simulink model "drones_simulation"  (R2025b)
settings: Solver=ode4  StartTime=0.0  StopTime=t_sim  FixedStep=Ts  RelTol=1e-3
values from neighbouring files (symbols this model uses):
  adj_row_1 = Adj_mat(1,:)    [Parameters_scenarios.m]
  adj_row_2 = Adj_mat(2,:)    [Parameters_scenarios.m]
  adj_row_3 = Adj_mat(3,:)    [Parameters_scenarios.m]
  adj_row_4 = Adj_mat(4,:)    [Parameters_scenarios.m]
  gamma1 = 8.0    (= 8)    [Parameters_scenarios.m]
  gamma2 = 8.0    (= 8)    [Parameters_scenarios.m]
  goal_tolerance = 0.05    [Parameters_scenarios.m]
  Ib = diag([Jxx, Jyy, Jzz])    [Parameters_scenarios.m]
  Kd = 2.5    [Parameters_scenarios.m]
  Kp = 1.2    [Parameters_scenarios.m]
  mass = 0.032    [Parameters_scenarios.m]
  max_acc = 2.5    [Parameters_scenarios.m]
  max_vel = 1.2 * (dist_total / desired_flight_time)    [Parameters_scenarios.m]
  Rc = 2.0    (= 2)    [Parameters_scenarios.m]
  Rs = Rs_safe    (= 0.15)    [Parameters_scenarios.m]
  Rs_obs = radius_robots + radii_obstacles + margin    (= 0.95)    [Parameters_scenarios.m]
  v0_1 = v0(1,:)'    [Parameters_scenarios.m]
  v0_2 = v0(2,:)'    [Parameters_scenarios.m]
  v0_3 = v0(3,:)'    [Parameters_scenarios.m]
  v0_4 = v0(4,:)'    [Parameters_scenarios.m]
  x0_1 = x0(1,:)'    [Parameters_scenarios.m]
  x0_2 = x0(2,:)'    [Parameters_scenarios.m]
  x0_3 = x0(3,:)'    [Parameters_scenarios.m]
  x0_4 = x0(4,:)'    [Parameters_scenarios.m]
  x_objects = [0.0 ... (first row only)    [Parameters_scenarios.m]
  xg_1 = xg(1,:)'    [Parameters_scenarios.m]
  xg_2 = xg(2,:)'    [Parameters_scenarios.m]
  xg_3 = xg(3,:)'    [Parameters_scenarios.m]
  xg_4 = xg(4,:)'    [Parameters_scenarios.m]
  xg_vec = reshape(xg', [], 1)    [Parameters_scenarios.m]
libraries: robotcorelib x4
(part 1 of 3)
settings Model: Creator=aless  LastModifiedBy=Alessia

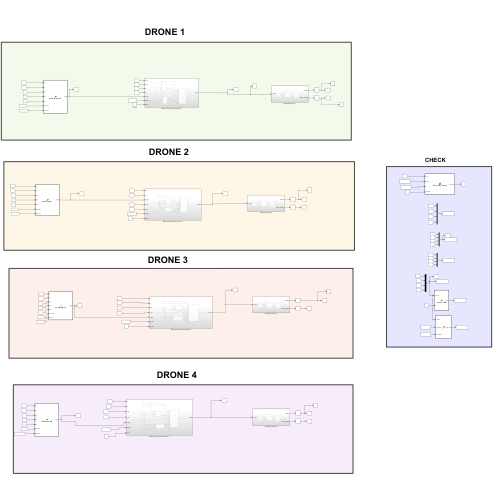
[thumbnail: Simulink's stored preview of the top-level diagram]
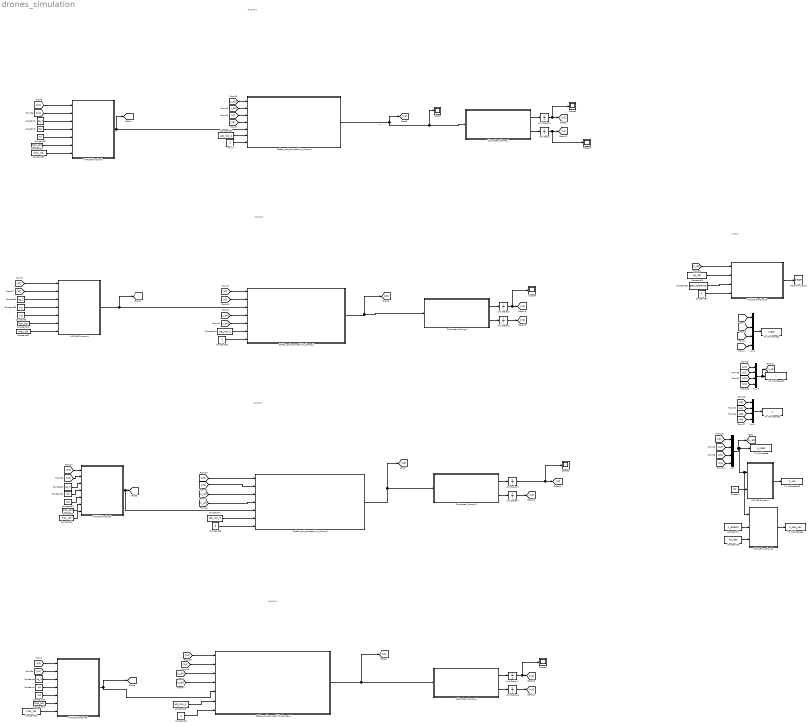
== system drones_simulation ==
  note: DRONE 1
  note: a
  note: DRONE 2
  note: DRONE 3
  note: DRONE 4
  note: CHECK
  Constant : Constant  Value=Rs
  Constant1 : Constant  Value=xg_1
  Constant17 : Constant  Value=x_objects
  Constant18 : Constant  Value=Rs_obs
  Constant2 : Constant  Value=xg_2
  Constant{6,27,32..33} (4 alike) : Constant  Value=Kd
  Constant{5,28..29,34} (4 alike) : Constant  Value=max_acc
  Constant3 : Constant  Value=xg_3
  Constant{4,7,30..31} (4 alike) : Constant  Value=Kp
  Constant47 : Constant  Value=adj_row_3
  Constant48 : Constant  Value=adj_row_4
  Constant49 : Constant  Value=adj_row_2
  Constant50 : Constant  Value=adj_row_1
  Constant52 : Constant  Value=2
  Constant53 : Constant  Value=3
  Constant54 : Constant  Value=4
  Constant{59..62} (4 alike) : Constant  Value=max_vel
  Constant63 : Constant  Value=goal_tolerance
  Constant64 : Constant  Value=4
  Constant65 : Constant  Value=xg_vec
  Constant8 : Constant  Value=xg_4
  MATLAB Function : MATLAB Function  TreatAsAtomicUnit=on
  MATLAB Function13 : MATLAB Function  TreatAsAtomicUnit=on
  MATLAB Function18 : MATLAB Function  TreatAsAtomicUnit=on
  MATLAB Function3 : MATLAB Function  TreatAsAtomicUnit=on
  MATLAB Function4 : MATLAB Function  TreatAsAtomicUnit=on
  MATLAB Function5 : MATLAB Function  TreatAsAtomicUnit=on
  MATLAB Function6 : MATLAB Function  TreatAsAtomicUnit=on
  Mux{,1..3} (4 alike) : Mux
  Safety_and_connectivity_Drone_1 : Subsystem
  Safety_and_connectivity_Drone_2 : Subsystem
  Safety_and_connectivity_Drone_3 : Subsystem
  Safety_and_connectivity_Drone_4 : Subsystem
  Scope{,3..7} (6 alike) : Scope
      Scope settings: ActiveDisplayYMinimum=-0.97415805527828381  ActiveDisplayYMaximum=3.2901969224528962
      Scope3 settings: ActiveDisplayYMinimum=-0.78272111630723207  ActiveDisplayYMaximum=1.9854335134906034  DataLoggingVariableName=ScopeData7
      Scope4 settings: ActiveDisplayYMinimum=-0.46546142132174678  ActiveDisplayYMaximum=0.18915279189572098  DataLoggingVariableName=ScopeData8
      Scope5 settings: ActiveDisplayYMinimum=-0.57335527047203139  ActiveDisplayYMaximum=1.160197434248283  DataLoggingVariableName=ScopeData9
      Scope6 settings: ActiveDisplayYMinimum=-0.5009829844423257  ActiveDisplayYMaximum=1.5088468599809324  DataLoggingVariableName=ScopeData10
      Scope7 settings: ActiveDisplayYMinimum=-0.78272111630723207  ActiveDisplayYMaximum=1.9854335134906034  DataLoggingVariableName=ScopeData12
  Stop Simulation : Stop
  Subsystem_Drone_1 : Subsystem
  Subsystem_Drone_2 : Subsystem
  Subsystem_Drone_3 : Subsystem
  Subsystem_Drone_4 : Subsystem
  To Workspace : ToWorkspace  VariableName=x_robot  SaveFormat=Timeseries  SampleTime=-1
  To Workspace1 : ToWorkspace  VariableName=u  SaveFormat=Timeseries  SampleTime=-1
  To Workspace2 : ToWorkspace  VariableName=u_gtg  SaveFormat=Timeseries  SampleTime=-1
  To Workspace3 : ToWorkspace  VariableName=h_vec  SaveFormat=Timeseries  SampleTime=-1
  To Workspace4 : ToWorkspace  VariableName=h_obs_vec  SaveFormat=Timeseries  SampleTime=-1
  To Workspace5 : ToWorkspace  VariableName=v  SaveFormat=Timeseries  SampleTime=-1
  Unit Delay{,1..7} (8 alike) : UnitDelay  SampleTime=-1  HasFrameUpgradeWarning=on
  my_id : Constant
  wires:
  [x4] -> Mux/4
  [x2] -> Mux/2
  [x4] -> MATLAB Function6/1(x_i)
  [x2] -> MATLAB Function4/1(x_i)
  Constant2/1 -> MATLAB Function4/3(xg_i)
  MATLAB Function/1(h_vec) -> To Workspace3/1
  Constant3/1 -> MATLAB Function5/3(xg_i)
  Mux1/1 -> To Workspace1/1
  Constant1/1 -> MATLAB Function3/3(xg_i)
  Mux/1 -> [x_all], To Workspace/1, MATLAB Function13/1(x_robot), MATLAB Function/1(x_robot)
  [x1] -> MATLAB Function3/1(x_i)
  [x1] -> Mux/1
  [u2] -> Mux1/2
  [x3] -> MATLAB Function5/1(x_i)
  [x3] -> Mux/3
  [u1] -> Mux1/1
  [u4] -> Mux1/4
  Constant/1 -> MATLAB Function/2(Rs)
  Constant8/1 -> MATLAB Function6/3(xg_i)
  [u3] -> Mux1/3
  Constant18/1 -> MATLAB Function13/3(Rs_objects)
  MATLAB Function13/1(h_obs_vec) -> To Workspace4/1
  Constant17/1 -> MATLAB Function13/2(x_objects)
  [u_gtg1] -> Mux2/1
  [u_gtg2] -> Mux2/2
  [u_gtg3] -> Mux2/3
  [u_gtg4] -> Mux2/4
  Mux2/1 -> To Workspace2/1
  [v3] -> Mux3/3
  Mux3/1 -> [v_all], To Workspace5/1
  [v1] -> Mux3/1
  [v2] -> Mux3/2
  [v4] -> Mux3/4
  [v1] -> MATLAB Function3/2(v_i)
  Constant7/1 -> MATLAB Function3/4(Kp)
  Constant27/1 -> MATLAB Function3/5(Kd)
  Constant28/1 -> MATLAB Function3/6(max_acc)
  [v2] -> MATLAB Function4/2(v_i)
  Constant29/1 -> MATLAB Function4/6(max_acc)
  Constant6/1 -> MATLAB Function4/5(Kd)
  Constant30/1 -> MATLAB Function4/4(Kp)
  [v3] -> MATLAB Function5/2(v_i)
  Constant31/1 -> MATLAB Function5/4(Kp)
  Constant32/1 -> MATLAB Function5/5(Kd)
  Constant5/1 -> MATLAB Function5/6(max_acc)
  Constant34/1 -> MATLAB Function6/6(max_acc)
  Constant33/1 -> MATLAB Function6/5(Kd)
  Constant4/1 -> MATLAB Function6/4(Kp)
  [v4] -> MATLAB Function6/2(v_i)
  MATLAB Function6/1(u_gtg) -> [u_gtg4], Safety_and_connectivity_Drone_4/5(u_gtg)
  MATLAB Function4/1(u_gtg) -> [u_gtg2], Safety_and_connectivity_Drone_2/3(u_gtg)
  Subsystem_Drone_1/1(Position) -> Unit Delay1/1
  Subsystem_Drone_1/2(Linear_velocity) -> Unit Delay/1
  Unit Delay1/1 -> Scope3/1, [x1]
  Unit Delay/1 -> Scope7/1, [v1]
  Unit Delay2/1 -> [v2]
  Subsystem_Drone_2/2(Linear_velocity) -> Unit Delay2/1
  Subsystem_Drone_2/1(Position) -> Unit Delay3/1
  Unit Delay4/1 -> [v3]
  Subsystem_Drone_3/2(Linear_velocity) -> Unit Delay4/1
  Subsystem_Drone_3/1(Position) -> Unit Delay5/1
  Unit Delay6/1 -> [v4]
  Subsystem_Drone_4/2(Linear_velocity) -> Unit Delay6/1
  Subsystem_Drone_4/1(Position) -> Unit Delay7/1
  Unit Delay3/1 -> Scope4/1, [x2]
  Unit Delay5/1 -> Scope5/1, [x3]
  Unit Delay7/1 -> Scope6/1, [x4]
  Constant59/1 -> MATLAB Function3/7(max_vel)
  Constant60/1 -> MATLAB Function4/7(max_vel)
  Constant61/1 -> MATLAB Function5/7(max_vel)
  Constant62/1 -> MATLAB Function6/7(max_vel)
  MATLAB Function18/1(stop_sim) -> Stop Simulation/1
  [x_all] -> MATLAB Function18/1(x_all)
  Constant63/1 -> MATLAB Function18/3(tol)
  Constant64/1 -> MATLAB Function18/4(n_robots)
  Constant65/1 -> MATLAB Function18/2(xg_vec)
  Safety_and_connectivity_Drone_1/1(u_safe) -> [u1], Scope/1, Subsystem_Drone_1/1(u_safe)
  MATLAB Function3/1(u_gtg) -> [u_gtg1], Safety_and_connectivity_Drone_1/5(u_gtg)
  Constant50/1 -> Safety_and_connectivity_Drone_1/6(adj_row)
  my_id/1 -> Safety_and_connectivity_Drone_1/7(my_id)
  [x_all] -> Safety_and_connectivity_Drone_1/1(x_all)
  [v_all] -> Safety_and_connectivity_Drone_1/2(v_all)
  [x1] -> Safety_and_connectivity_Drone_1/3(x_i)
  [v1] -> Safety_and_connectivity_Drone_1/4(v_i)
  Safety_and_connectivity_Drone_2/1(u_safe) -> [u2], Subsystem_Drone_2/1(u_safe)
  [x2] -> Safety_and_connectivity_Drone_2/1(x_i)
  [v2] -> Safety_and_connectivity_Drone_2/2(v_i)
  [x_all] -> Safety_and_connectivity_Drone_2/4(x_all)
  [v_all] -> Safety_and_connectivity_Drone_2/5(v_all)
  Constant49/1 -> Safety_and_connectivity_Drone_2/6(adj_row)
  Constant52/1 -> Safety_and_connectivity_Drone_2/7(my_id)
  Safety_and_connectivity_Drone_3/1(u_safe) -> [u3], Subsystem_Drone_3/1(u_safe)
  [x3] -> Safety_and_connectivity_Drone_3/1(x_i)
  [v3] -> Safety_and_connectivity_Drone_3/2(v_i)
  [x_all] -> Safety_and_connectivity_Drone_3/3(x_all)
  [v_all] -> Safety_and_connectivity_Drone_3/4(v_all)
  MATLAB Function5/1(u_gtg) -> Safety_and_connectivity_Drone_3/5(u_gtg), [u_gtg3]
  Constant47/1 -> Safety_and_connectivity_Drone_3/6(adj_row)
  Constant53/1 -> Safety_and_connectivity_Drone_3/7(my_id)
  Safety_and_connectivity_Drone_4/1(u_safe) -> [u4], Subsystem_Drone_4/1(u_safe)
  [x4] -> Safety_and_connectivity_Drone_4/1(x_i)
  [v4] -> Safety_and_connectivity_Drone_4/2(v_i)
  [x_all] -> Safety_and_connectivity_Drone_4/3(x_all)
  [v_all] -> Safety_and_connectivity_Drone_4/4(v_all)
  Constant48/1 -> Safety_and_connectivity_Drone_4/6(adj_row)
  Constant54/1 -> Safety_and_connectivity_Drone_4/7(my_id)

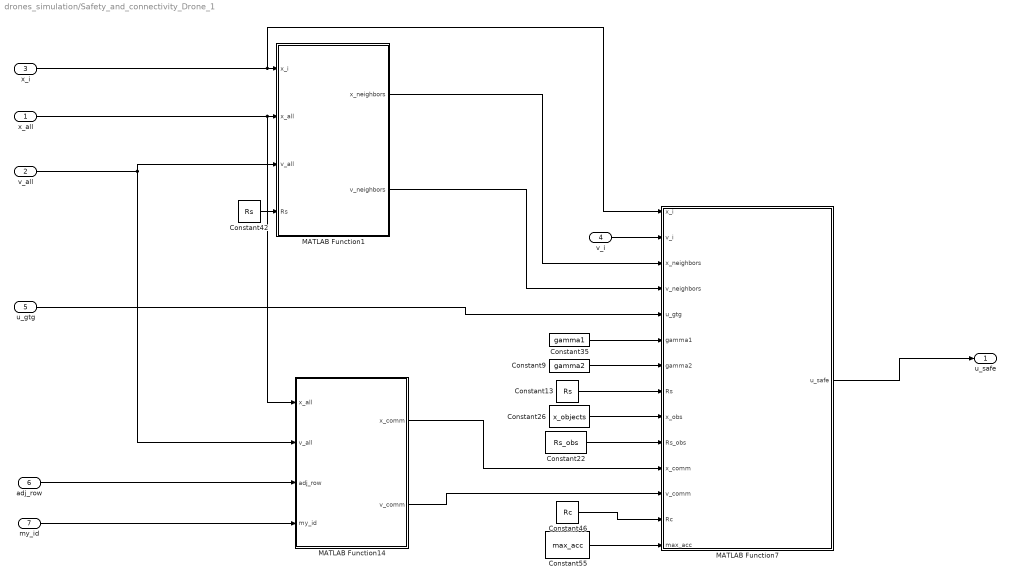
== system drones_simulation/Safety_and_connectivity_Drone_1 ==
  x_all : Inport
  v_all : Inport  Port=2
  x_i : Inport  Port=3
  v_i : Inport  Port=4
  u_gtg : Inport  Port=5
  adj_row : Inport  Port=6
  my_id : Inport  Port=7
  Constant13 : Constant  Value=Rs
  Constant22 : Constant  Value=Rs_obs
  Constant26 : Constant  Value=x_objects
  Constant35 : Constant  Value=gamma1
  Constant42 : Constant  Value=Rs
  Constant46 : Constant  Value=Rc
  Constant55 : Constant  Value=max_acc
  Constant9 : Constant  Value=gamma2
  MATLAB Function1 : MATLAB Function  TreatAsAtomicUnit=on
  MATLAB Function14 : MATLAB Function  TreatAsAtomicUnit=on
  MATLAB Function7 : MATLAB Function  TreatAsAtomicUnit=on
  u_safe : Outport
  wires:
  Constant35/1 -> MATLAB Function7/6(gamma1)
  Constant42/1 -> MATLAB Function1/4(Rs)
  u_gtg/1 -> MATLAB Function7/5(u_gtg)
  Constant22/1 -> MATLAB Function7/10(Rs_obs)
  Constant26/1 -> MATLAB Function7/9(x_obs)
  Constant55/1 -> MATLAB Function7/14(max_acc)
  MATLAB Function1/2(v_neighbors) -> MATLAB Function7/4(v_neighbors)
  MATLAB Function14/2(v_comm) -> MATLAB Function7/12(v_comm)
  MATLAB Function1/1(x_neighbors) -> MATLAB Function7/3(x_neighbors)
  MATLAB Function14/1(x_comm) -> MATLAB Function7/11(x_comm)
  Constant13/1 -> MATLAB Function7/8(Rs)
  x_all/1 -> MATLAB Function14/1(x_all), MATLAB Function1/2(x_all)
  Constant46/1 -> MATLAB Function7/13(Rc)
  Constant9/1 -> MATLAB Function7/7(gamma2)
  v_all/1 -> MATLAB Function1/3(v_all), MATLAB Function14/2(v_all)
  adj_row/1 -> MATLAB Function14/3(adj_row)
  MATLAB Function7/1(u_safe) -> u_safe/1
  my_id/1 -> MATLAB Function14/4(my_id)
  x_i/1 -> MATLAB Function7/1(x_i), MATLAB Function1/1(x_i)
  v_i/1 -> MATLAB Function7/2(v_i)

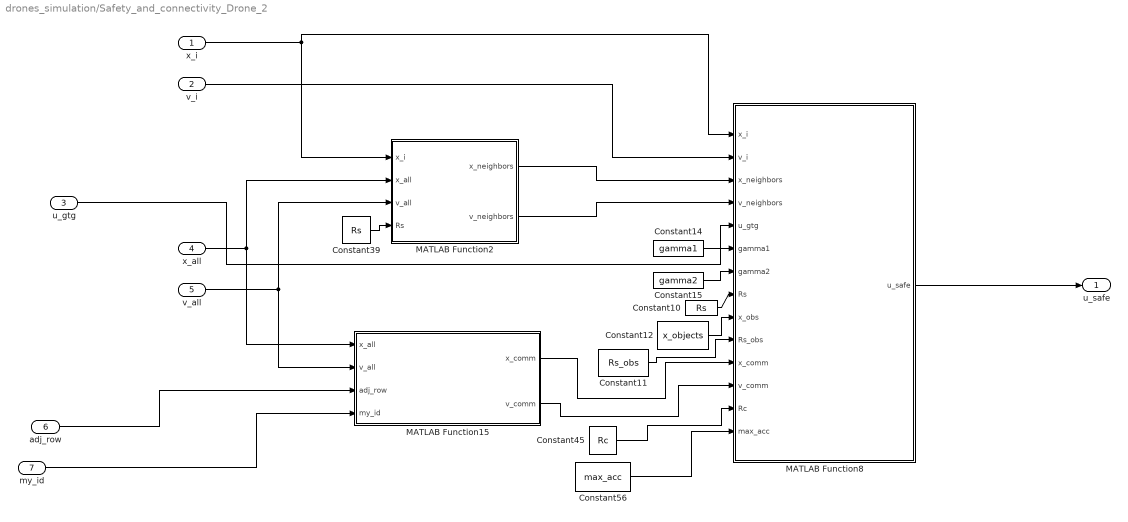
== system drones_simulation/Safety_and_connectivity_Drone_2 ==
  x_i : Inport
  v_i : Inport  Port=2
  u_gtg : Inport  Port=3
  x_all : Inport  Port=4
  v_all : Inport  Port=5
  adj_row : Inport  Port=6
  my_id : Inport  Port=7
  Constant10 : Constant  Value=Rs
  Constant11 : Constant  Value=Rs_obs
  Constant12 : Constant  Value=x_objects
  Constant14 : Constant  Value=gamma1
  Constant15 : Constant  Value=gamma2
  Constant39 : Constant  Value=Rs
  Constant45 : Constant  Value=Rc
  Constant56 : Constant  Value=max_acc
  MATLAB Function15 : MATLAB Function  TreatAsAtomicUnit=on
  MATLAB Function2 : MATLAB Function  TreatAsAtomicUnit=on
  MATLAB Function8 : MATLAB Function  TreatAsAtomicUnit=on
  u_safe : Outport
  wires:
  MATLAB Function2/2(v_neighbors) -> MATLAB Function8/4(v_neighbors)
  Constant39/1 -> MATLAB Function2/4(Rs)
  Constant45/1 -> MATLAB Function8/13(Rc)
  MATLAB Function2/1(x_neighbors) -> MATLAB Function8/3(x_neighbors)
  MATLAB Function15/2(v_comm) -> MATLAB Function8/12(v_comm)
  MATLAB Function15/1(x_comm) -> MATLAB Function8/11(x_comm)
  x_i/1 -> MATLAB Function2/1(x_i), MATLAB Function8/1(x_i)
  Constant10/1 -> MATLAB Function8/8(Rs)
  Constant15/1 -> MATLAB Function8/7(gamma2)
  Constant12/1 -> MATLAB Function8/9(x_obs)
  v_all/1 -> MATLAB Function15/2(v_all), MATLAB Function2/3(v_all)
  Constant14/1 -> MATLAB Function8/6(gamma1)
  Constant11/1 -> MATLAB Function8/10(Rs_obs)
  Constant56/1 -> MATLAB Function8/14(max_acc)
  x_all/1 -> MATLAB Function15/1(x_all), MATLAB Function2/2(x_all)
  adj_row/1 -> MATLAB Function15/3(adj_row)
  u_gtg/1 -> MATLAB Function8/5(u_gtg)
  my_id/1 -> MATLAB Function15/4(my_id)
  v_i/1 -> MATLAB Function8/2(v_i)
  MATLAB Function8/1(u_safe) -> u_safe/1

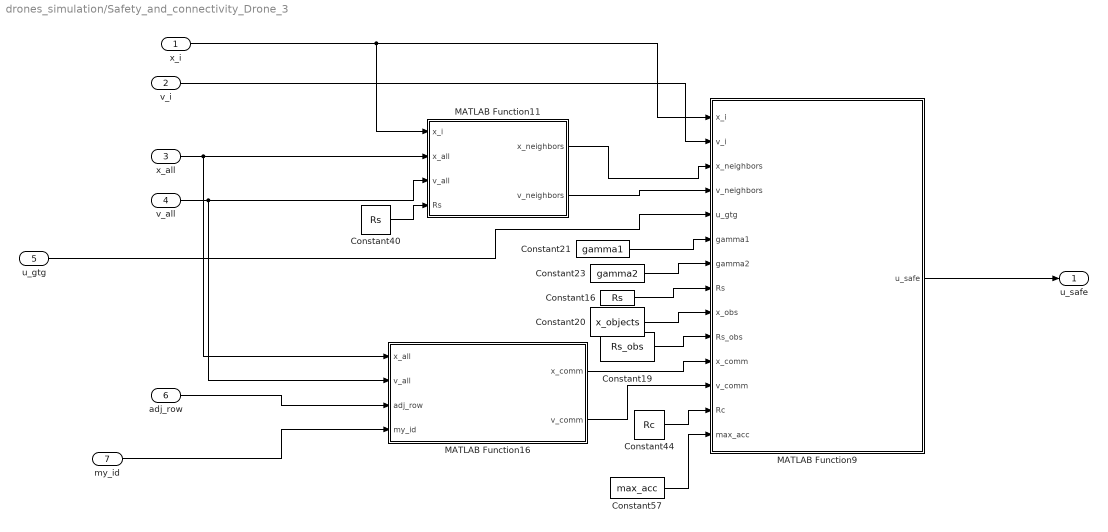
== system drones_simulation/Safety_and_connectivity_Drone_3 ==
  x_i : Inport
  v_i : Inport  Port=2
  x_all : Inport  Port=3
  v_all : Inport  Port=4
  u_gtg : Inport  Port=5
  adj_row : Inport  Port=6
  my_id : Inport  Port=7
  Constant16 : Constant  Value=Rs
  Constant19 : Constant  Value=Rs_obs
  Constant20 : Constant  Value=x_objects
  Constant21 : Constant  Value=gamma1
  Constant23 : Constant  Value=gamma2
  Constant40 : Constant  Value=Rs
  Constant44 : Constant  Value=Rc
  Constant57 : Constant  Value=max_acc
  MATLAB Function11 : MATLAB Function  TreatAsAtomicUnit=on
  MATLAB Function16 : MATLAB Function  TreatAsAtomicUnit=on
  MATLAB Function9 : MATLAB Function  TreatAsAtomicUnit=on
  u_safe : Outport
  wires:
  MATLAB Function11/2(v_neighbors) -> MATLAB Function9/4(v_neighbors)
  v_all/1 -> MATLAB Function11/3(v_all), MATLAB Function16/2(v_all)
  MATLAB Function16/1(x_comm) -> MATLAB Function9/11(x_comm)
  Constant20/1 -> MATLAB Function9/9(x_obs)
  Constant16/1 -> MATLAB Function9/8(Rs)
  v_i/1 -> MATLAB Function9/2(v_i)
  Constant40/1 -> MATLAB Function11/4(Rs)
  Constant23/1 -> MATLAB Function9/7(gamma2)
  u_gtg/1 -> MATLAB Function9/5(u_gtg)
  Constant57/1 -> MATLAB Function9/14(max_acc)
  Constant21/1 -> MATLAB Function9/6(gamma1)
  MATLAB Function11/1(x_neighbors) -> MATLAB Function9/3(x_neighbors)
  x_all/1 -> MATLAB Function11/2(x_all), MATLAB Function16/1(x_all)
  Constant44/1 -> MATLAB Function9/13(Rc)
  Constant19/1 -> MATLAB Function9/10(Rs_obs)
  MATLAB Function16/2(v_comm) -> MATLAB Function9/12(v_comm)
  x_i/1 -> MATLAB Function9/1(x_i), MATLAB Function11/1(x_i)
  adj_row/1 -> MATLAB Function16/3(adj_row)
  my_id/1 -> MATLAB Function16/4(my_id)
  MATLAB Function9/1(u_safe) -> u_safe/1

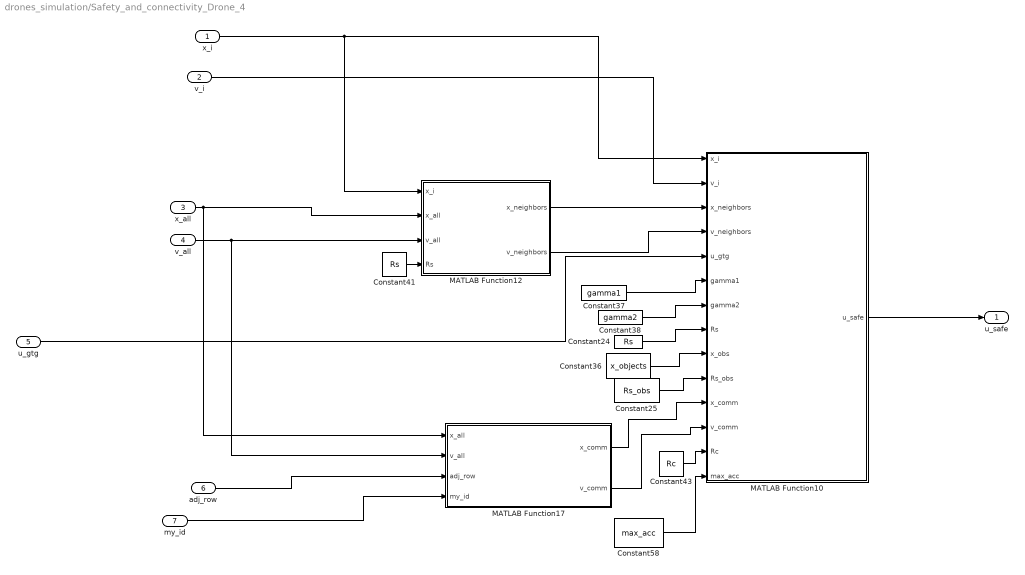
== system drones_simulation/Safety_and_connectivity_Drone_4 ==
  x_i : Inport
  v_i : Inport  Port=2
  x_all : Inport  Port=3
  v_all : Inport  Port=4
  u_gtg : Inport  Port=5
  adj_row : Inport  Port=6
  my_id : Inport  Port=7
  Constant24 : Constant  Value=Rs
  Constant25 : Constant  Value=Rs_obs
  Constant36 : Constant  Value=x_objects
  Constant37 : Constant  Value=gamma1
  Constant38 : Constant  Value=gamma2
  Constant41 : Constant  Value=Rs
  Constant43 : Constant  Value=Rc
  Constant58 : Constant  Value=max_acc
  MATLAB Function10 : MATLAB Function  TreatAsAtomicUnit=on
  MATLAB Function12 : MATLAB Function  TreatAsAtomicUnit=on
  MATLAB Function17 : MATLAB Function  TreatAsAtomicUnit=on
  u_safe : Outport
  wires:
  x_all/1 -> MATLAB Function17/1(x_all), MATLAB Function12/2(x_all)
  MATLAB Function12/2(v_neighbors) -> MATLAB Function10/4(v_neighbors)
  Constant58/1 -> MATLAB Function10/14(max_acc)
  Constant25/1 -> MATLAB Function10/10(Rs_obs)
  adj_row/1 -> MATLAB Function17/3(adj_row)
  Constant38/1 -> MATLAB Function10/7(gamma2)
  Constant43/1 -> MATLAB Function10/13(Rc)
  MATLAB Function12/1(x_neighbors) -> MATLAB Function10/3(x_neighbors)
  MATLAB Function17/1(x_comm) -> MATLAB Function10/11(x_comm)
  MATLAB Function17/2(v_comm) -> MATLAB Function10/12(v_comm)
  Constant36/1 -> MATLAB Function10/9(x_obs)
  Constant37/1 -> MATLAB Function10/6(gamma1)
  Constant41/1 -> MATLAB Function12/4(Rs)
  u_gtg/1 -> MATLAB Function10/5(u_gtg)
  Constant24/1 -> MATLAB Function10/8(Rs)
  x_i/1 -> MATLAB Function10/1(x_i), MATLAB Function12/1(x_i)
  v_all/1 -> MATLAB Function17/2(v_all), MATLAB Function12/3(v_all)
  MATLAB Function10/1(u_safe) -> u_safe/1
  v_i/1 -> MATLAB Function10/2(v_i)
  my_id/1 -> MATLAB Function17/4(my_id)

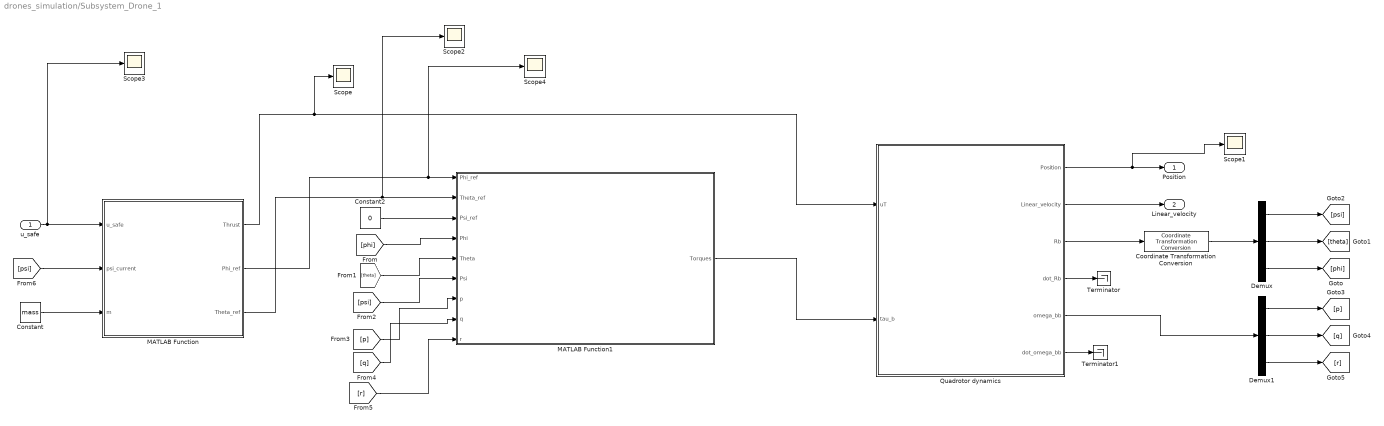
== system drones_simulation/Subsystem_Drone_1 ==
  u_safe : Inport
  Constant : Constant  Value=mass
  Constant2 : Constant  Value=0
  Coordinate Transformation Conversion : robotcorelib/Coordinate Transformation Conversion  InputRepresentation=Rotation Matrix  InputEulerSequence=ZYX  ShowTrVecInputPort=on  OutputRepresentation=Euler Angles  OutputEulerSequence=ZYX  ShowTrVecOutputPort=on  SimulateUsing=Interpreted execution
  Demux : Demux  Outputs=3
  Demux1 : Demux  Outputs=3
  MATLAB Function : MATLAB Function  TreatAsAtomicUnit=on
  MATLAB Function1 : MATLAB Function  TreatAsAtomicUnit=on
  Quadrotor dynamics : Subsystem
  Scope{,1..4} (5 alike) : Scope
      Scope settings: ActiveDisplayYMinimum=0.23486779023141996  ActiveDisplayYMaximum=0.45370086939324927
      Scope1 settings: ActiveDisplayYMinimum=-1  ActiveDisplayYMaximum=1  DataLoggingVariableName=ScopeData4
      Scope2 settings: ActiveDisplayYMinimum=-0.029456486854581094  ActiveDisplayYMaximum=0.010266383729965845  DataLoggingVariableName=ScopeData5
      Scope3 settings: ActiveDisplayYMinimum=-0.584568773397757  ActiveDisplayYMaximum=0.56237356855011467  DataLoggingVariableName=ScopeData6
      Scope4 settings: ActiveDisplayYMinimum=-0.10558082577098628  ActiveDisplayYMaximum=0.03279467874545524  DataLoggingVariableName=ScopeData11
  Terminator : Terminator
  Terminator1 : Terminator
  Position : Outport
  Linear_velocity : Outport  Port=2
  wires:
  u_safe/1 -> Scope3/1, MATLAB Function/1(u_safe)
  Constant/1 -> MATLAB Function/3(m)
  [psi] -> MATLAB Function/2(psi_current)
  MATLAB Function/2(Phi_ref) -> Scope4/1, MATLAB Function1/1(Phi_ref)
  MATLAB Function/3(Theta_ref) -> Scope2/1, MATLAB Function1/2(Theta_ref)
  Constant2/1 -> MATLAB Function1/3(Psi_ref)
  Quadrotor dynamics/3(Rb) -> Coordinate Transformation Conversion/1
  MATLAB Function/1(Thrust) -> Scope/1, Quadrotor dynamics/1(uT)
  MATLAB Function1/1(Torques) -> Quadrotor dynamics/2(tau_b)
  Coordinate Transformation Conversion/1 -> Demux/1
  Demux/2 -> [theta]
  [phi] -> MATLAB Function1/4(Phi)
  [theta] -> MATLAB Function1/5(Theta)
  [psi] -> MATLAB Function1/6(Psi)
  Demux1/3 -> [r]
  Demux1/2 -> [q]
  Demux1/1 -> [p]
  Quadrotor dynamics/5(omega_bb) -> Demux1/1
  [p] -> MATLAB Function1/7(p)
  [q] -> MATLAB Function1/8(q)
  [r] -> MATLAB Function1/9(r)
  Quadrotor dynamics/1(Position) -> Scope1/1, Position/1
  Quadrotor dynamics/2(Linear_velocity) -> Linear_velocity/1
  Quadrotor dynamics/4(dot_Rb) -> Terminator/1
  Quadrotor dynamics/6(dot_omega_bb) -> Terminator1/1
  Demux/1 -> [psi]
  Demux/3 -> [phi]

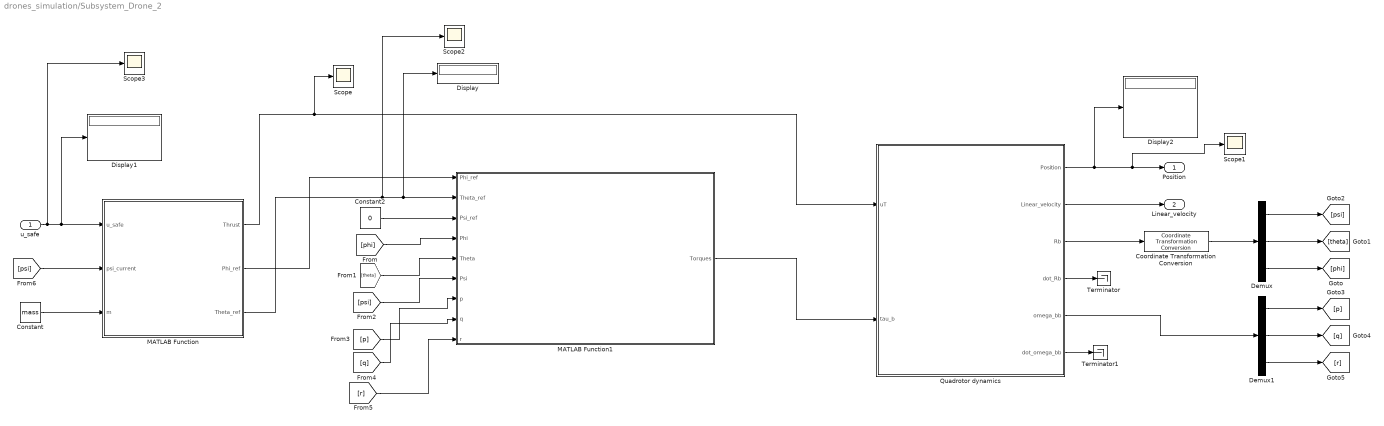
== system drones_simulation/Subsystem_Drone_2 ==
  u_safe : Inport
  Constant : Constant  Value=mass
  Constant2 : Constant  Value=0
  Coordinate Transformation Conversion : robotcorelib/Coordinate Transformation Conversion  InputRepresentation=Rotation Matrix  InputEulerSequence=ZYX  ShowTrVecInputPort=on  OutputRepresentation=Euler Angles  OutputEulerSequence=ZYX  ShowTrVecOutputPort=on  SimulateUsing=Interpreted execution
  Demux : Demux  Outputs=3
  Demux1 : Demux  Outputs=3
  Display : Display
  Display1 : Display
  Display2 : Display
  MATLAB Function : MATLAB Function  TreatAsAtomicUnit=on
  MATLAB Function1 : MATLAB Function  TreatAsAtomicUnit=on
  Quadrotor dynamics : Subsystem
  Scope{,1..3} (4 alike) : Scope
      Scope settings: ActiveDisplayYMinimum=0.23486779023141996  ActiveDisplayYMaximum=0.45370086939324927
      Scope1 settings: ActiveDisplayYMinimum=-1  ActiveDisplayYMaximum=1  DataLoggingVariableName=ScopeData4
      Scope2 settings: ActiveDisplayYMinimum=-0.036348339933849928  ActiveDisplayYMaximum=0.031372766654044378  DataLoggingVariableName=ScopeData5
      Scope3 settings: ActiveDisplayYMinimum=-0.584568773397757  ActiveDisplayYMaximum=0.56237356855011467  DataLoggingVariableName=ScopeData6
  Terminator : Terminator
  Terminator1 : Terminator
  Position : Outport
  Linear_velocity : Outport  Port=2
  wires:
  u_safe/1 -> Scope3/1, Display1/1, MATLAB Function/1(u_safe)
  Constant/1 -> MATLAB Function/3(m)
  [psi] -> MATLAB Function/2(psi_current)
  MATLAB Function/2(Phi_ref) -> MATLAB Function1/1(Phi_ref)
  MATLAB Function/3(Theta_ref) -> Scope2/1, Display/1, MATLAB Function1/2(Theta_ref)
  Constant2/1 -> MATLAB Function1/3(Psi_ref)
  Quadrotor dynamics/3(Rb) -> Coordinate Transformation Conversion/1
  MATLAB Function/1(Thrust) -> Scope/1, Quadrotor dynamics/1(uT)
  MATLAB Function1/1(Torques) -> Quadrotor dynamics/2(tau_b)
  Coordinate Transformation Conversion/1 -> Demux/1
  Demux/2 -> [theta]
  [phi] -> MATLAB Function1/4(Phi)
  [theta] -> MATLAB Function1/5(Theta)
  [psi] -> MATLAB Function1/6(Psi)
  Demux1/3 -> [r]
  Demux1/2 -> [q]
  Demux1/1 -> [p]
  Quadrotor dynamics/5(omega_bb) -> Demux1/1
  [p] -> MATLAB Function1/7(p)
  [q] -> MATLAB Function1/8(q)
  [r] -> MATLAB Function1/9(r)
  Quadrotor dynamics/1(Position) -> Display2/1, Scope1/1, Position/1
  Quadrotor dynamics/2(Linear_velocity) -> Linear_velocity/1
  Quadrotor dynamics/4(dot_Rb) -> Terminator/1
  Quadrotor dynamics/6(dot_omega_bb) -> Terminator1/1
  Demux/1 -> [psi]
  Demux/3 -> [phi]

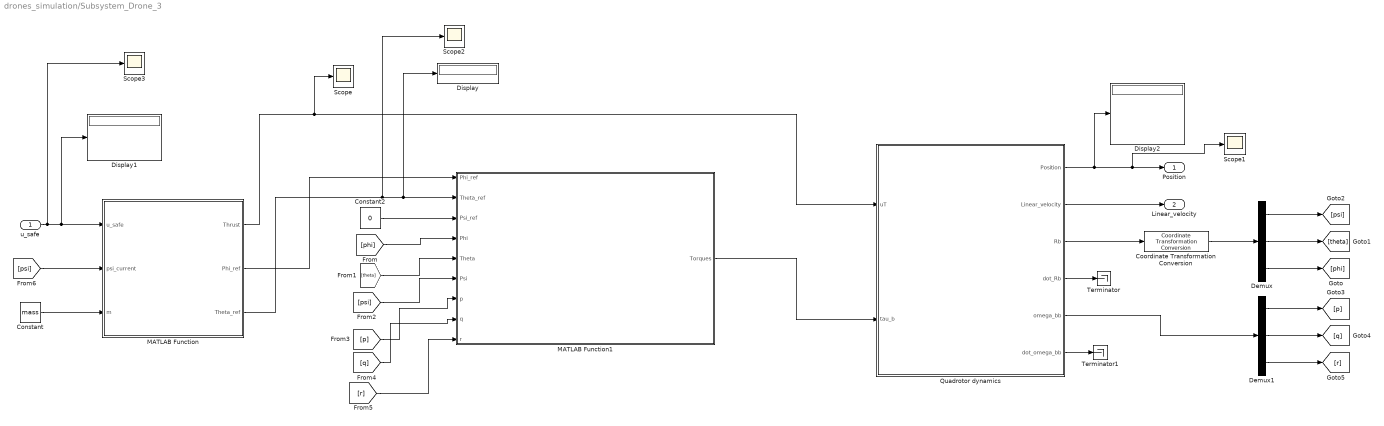
== system drones_simulation/Subsystem_Drone_3 ==
  u_safe : Inport
  Constant : Constant  Value=mass
  Constant2 : Constant  Value=0
  Coordinate Transformation Conversion : robotcorelib/Coordinate Transformation Conversion  InputRepresentation=Rotation Matrix  InputEulerSequence=ZYX  ShowTrVecInputPort=on  OutputRepresentation=Euler Angles  OutputEulerSequence=ZYX  ShowTrVecOutputPort=on  SimulateUsing=Interpreted execution
  Demux : Demux  Outputs=3
  Demux1 : Demux  Outputs=3
  Display : Display
  Display1 : Display
  Display2 : Display
  MATLAB Function : MATLAB Function  TreatAsAtomicUnit=on
  MATLAB Function1 : MATLAB Function  TreatAsAtomicUnit=on
  Quadrotor dynamics : Subsystem
  Scope{,1..3} (4 alike) : Scope
      Scope settings: ActiveDisplayYMinimum=0.23486779023141996  ActiveDisplayYMaximum=0.45370086939324927
      Scope1 settings: ActiveDisplayYMinimum=-0.78202717260171462  ActiveDisplayYMaximum=1.9952624356819166  DataLoggingVariableName=ScopeData4
      Scope2 settings: ActiveDisplayYMinimum=-0.036348339933849928  ActiveDisplayYMaximum=0.031372766654044378  DataLoggingVariableName=ScopeData5
      Scope3 settings: ActiveDisplayYMinimum=-0.584568773397757  ActiveDisplayYMaximum=0.56237356855011467  DataLoggingVariableName=ScopeData6
  Terminator : Terminator
  Terminator1 : Terminator
  Position : Outport
  Linear_velocity : Outport  Port=2
  wires:
  u_safe/1 -> Scope3/1, Display1/1, MATLAB Function/1(u_safe)
  Constant/1 -> MATLAB Function/3(m)
  [psi] -> MATLAB Function/2(psi_current)
  MATLAB Function/2(Phi_ref) -> MATLAB Function1/1(Phi_ref)
  MATLAB Function/3(Theta_ref) -> Scope2/1, Display/1, MATLAB Function1/2(Theta_ref)
  Constant2/1 -> MATLAB Function1/3(Psi_ref)
  Quadrotor dynamics/3(Rb) -> Coordinate Transformation Conversion/1
  MATLAB Function/1(Thrust) -> Scope/1, Quadrotor dynamics/1(uT)
  MATLAB Function1/1(Torques) -> Quadrotor dynamics/2(tau_b)
  Coordinate Transformation Conversion/1 -> Demux/1
  Demux/2 -> [theta]
  [phi] -> MATLAB Function1/4(Phi)
  [theta] -> MATLAB Function1/5(Theta)
  [psi] -> MATLAB Function1/6(Psi)
  Demux1/3 -> [r]
  Demux1/2 -> [q]
  Demux1/1 -> [p]
  Quadrotor dynamics/5(omega_bb) -> Demux1/1
  [p] -> MATLAB Function1/7(p)
  [q] -> MATLAB Function1/8(q)
  [r] -> MATLAB Function1/9(r)
  Quadrotor dynamics/1(Position) -> Display2/1, Scope1/1, Position/1
  Quadrotor dynamics/2(Linear_velocity) -> Linear_velocity/1
  Quadrotor dynamics/4(dot_Rb) -> Terminator/1
  Quadrotor dynamics/6(dot_omega_bb) -> Terminator1/1
  Demux/1 -> [psi]
  Demux/3 -> [phi]

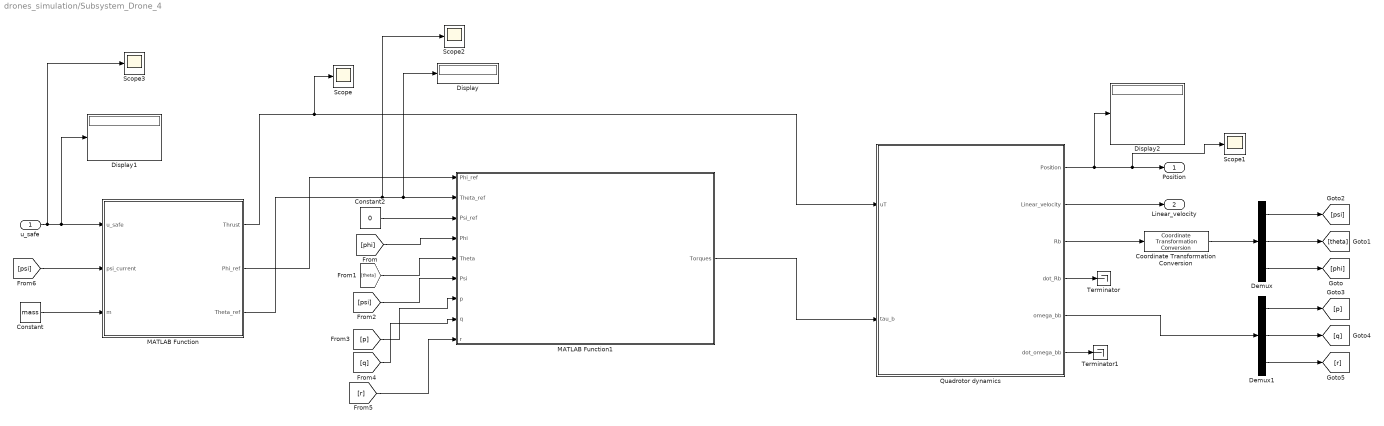
== system drones_simulation/Subsystem_Drone_4 ==
  u_safe : Inport
  Constant : Constant  Value=mass
  Constant2 : Constant  Value=0
  Coordinate Transformation Conversion : robotcorelib/Coordinate Transformation Conversion  InputRepresentation=Rotation Matrix  InputEulerSequence=ZYX  ShowTrVecInputPort=on  OutputRepresentation=Euler Angles  OutputEulerSequence=ZYX  ShowTrVecOutputPort=on  SimulateUsing=Interpreted execution
  Demux : Demux  Outputs=3
  Demux1 : Demux  Outputs=3
  Display : Display
  Display1 : Display
  Display2 : Display
  MATLAB Function : MATLAB Function  TreatAsAtomicUnit=on
  MATLAB Function1 : MATLAB Function  TreatAsAtomicUnit=on
  Quadrotor dynamics : Subsystem
  Scope{,1..3} (4 alike) : Scope
      Scope settings: ActiveDisplayYMinimum=0.23486779023141996  ActiveDisplayYMaximum=0.45370086939324927
      Scope1 settings: ActiveDisplayYMinimum=-0.78202717260171462  ActiveDisplayYMaximum=1.9952624356819166  DataLoggingVariableName=ScopeData4
      Scope2 settings: ActiveDisplayYMinimum=-0.036348339933849928  ActiveDisplayYMaximum=0.031372766654044378  DataLoggingVariableName=ScopeData5
      Scope3 settings: ActiveDisplayYMinimum=-0.584568773397757  ActiveDisplayYMaximum=0.56237356855011467  DataLoggingVariableName=ScopeData6
  Terminator : Terminator
  Terminator1 : Terminator
  Position : Outport
  Linear_velocity : Outport  Port=2
  wires:
  u_safe/1 -> Scope3/1, Display1/1, MATLAB Function/1(u_safe)
  Constant/1 -> MATLAB Function/3(m)
  [psi] -> MATLAB Function/2(psi_current)
  MATLAB Function/2(Phi_ref) -> MATLAB Function1/1(Phi_ref)
  MATLAB Function/3(Theta_ref) -> Scope2/1, Display/1, MATLAB Function1/2(Theta_ref)
  Constant2/1 -> MATLAB Function1/3(Psi_ref)
  Quadrotor dynamics/3(Rb) -> Coordinate Transformation Conversion/1
  MATLAB Function/1(Thrust) -> Scope/1, Quadrotor dynamics/1(uT)
  MATLAB Function1/1(Torques) -> Quadrotor dynamics/2(tau_b)
  Coordinate Transformation Conversion/1 -> Demux/1
  Demux/2 -> [theta]
  [phi] -> MATLAB Function1/4(Phi)
  [theta] -> MATLAB Function1/5(Theta)
  [psi] -> MATLAB Function1/6(Psi)
  Demux1/3 -> [r]
  Demux1/2 -> [q]
  Demux1/1 -> [p]
  Quadrotor dynamics/5(omega_bb) -> Demux1/1
  [p] -> MATLAB Function1/7(p)
  [q] -> MATLAB Function1/8(q)
  [r] -> MATLAB Function1/9(r)
  Quadrotor dynamics/1(Position) -> Display2/1, Scope1/1, Position/1
  Quadrotor dynamics/2(Linear_velocity) -> Linear_velocity/1
  Quadrotor dynamics/4(dot_Rb) -> Terminator/1
  Quadrotor dynamics/6(dot_omega_bb) -> Terminator1/1
  Demux/1 -> [psi]
  Demux/3 -> [phi]

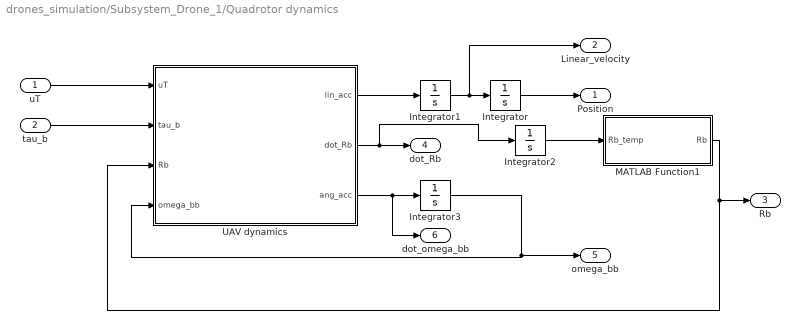
== system drones_simulation/Subsystem_Drone_1/Quadrotor dynamics ==
  uT : Inport
  tau_b : Inport  Port=2
  Integrator : Integrator  InitialCondition=x0_1
  Integrator1 : Integrator  InitialCondition=v0_1
  Integrator2 : Integrator  InitialCondition=[1 0 0; 0 1 0;0 0 1]
  Integrator3 : Integrator  InitialCondition=[0;0;0]
  MATLAB Function1 : MATLAB Function  TreatAsAtomicUnit=on
  UAV dynamics : MATLAB Function  TreatAsAtomicUnit=on
  Position : Outport
  Linear_velocity : Outport  Port=2
  Rb : Outport  Port=3
  dot_Rb : Outport  Port=4
  omega_bb : Outport  Port=5
  dot_omega_bb : Outport  Port=6
  wires:
  tau_b/1 -> UAV dynamics/2(tau_b)
  Integrator/1 -> Position/1
  UAV dynamics/3(ang_acc) -> dot_omega_bb/1, Integrator3/1
  UAV dynamics/1(lin_acc) -> Integrator1/1
  uT/1 -> UAV dynamics/1(uT)
  Integrator1/1 -> Linear_velocity/1, Integrator/1
  Integrator3/1 -> UAV dynamics/4(omega_bb), omega_bb/1
  UAV dynamics/2(dot_Rb) -> Integrator2/1, dot_Rb/1
  MATLAB Function1/1(Rb) -> Rb/1, UAV dynamics/3(Rb)
  Integrator2/1 -> MATLAB Function1/1(Rb_temp)

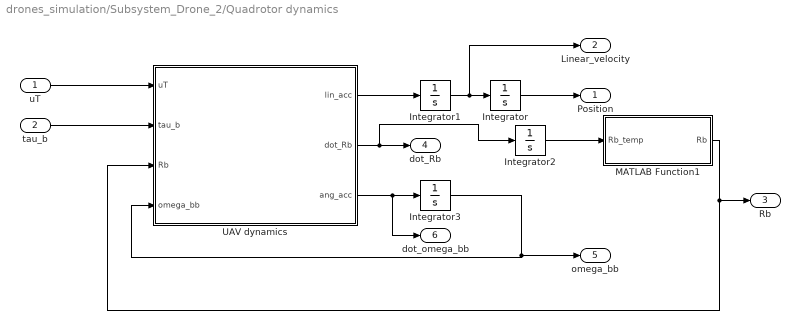
== system drones_simulation/Subsystem_Drone_2/Quadrotor dynamics ==
  uT : Inport
  tau_b : Inport  Port=2
  Integrator : Integrator  InitialCondition=x0_2
  Integrator1 : Integrator  InitialCondition=v0_2
  Integrator2 : Integrator  InitialCondition=[1 0 0; 0 1 0;0 0 1]
  Integrator3 : Integrator  InitialCondition=[0;0;0]
  MATLAB Function1 : MATLAB Function  TreatAsAtomicUnit=on
  UAV dynamics : MATLAB Function  TreatAsAtomicUnit=on
  Position : Outport
  Linear_velocity : Outport  Port=2
  Rb : Outport  Port=3
  dot_Rb : Outport  Port=4
  omega_bb : Outport  Port=5
  dot_omega_bb : Outport  Port=6
  wires:
  tau_b/1 -> UAV dynamics/2(tau_b)
  Integrator/1 -> Position/1
  UAV dynamics/3(ang_acc) -> dot_omega_bb/1, Integrator3/1
  UAV dynamics/1(lin_acc) -> Integrator1/1
  uT/1 -> UAV dynamics/1(uT)
  Integrator1/1 -> Linear_velocity/1, Integrator/1
  Integrator3/1 -> UAV dynamics/4(omega_bb), omega_bb/1
  UAV dynamics/2(dot_Rb) -> Integrator2/1, dot_Rb/1
  MATLAB Function1/1(Rb) -> Rb/1, UAV dynamics/3(Rb)
  Integrator2/1 -> MATLAB Function1/1(Rb_temp)

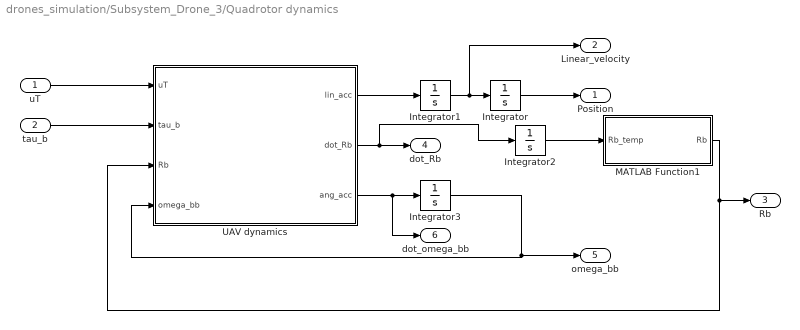
== system drones_simulation/Subsystem_Drone_3/Quadrotor dynamics ==
  uT : Inport
  tau_b : Inport  Port=2
  Integrator : Integrator  InitialCondition=x0_3
  Integrator1 : Integrator  InitialCondition=v0_3
  Integrator2 : Integrator  InitialCondition=[1 0 0; 0 1 0;0 0 1]
  Integrator3 : Integrator  InitialCondition=[0;0;0]
  MATLAB Function1 : MATLAB Function  TreatAsAtomicUnit=on
  UAV dynamics : MATLAB Function  TreatAsAtomicUnit=on
  Position : Outport
  Linear_velocity : Outport  Port=2
  Rb : Outport  Port=3
  dot_Rb : Outport  Port=4
  omega_bb : Outport  Port=5
  dot_omega_bb : Outport  Port=6
  wires:
  tau_b/1 -> UAV dynamics/2(tau_b)
  Integrator/1 -> Position/1
  UAV dynamics/3(ang_acc) -> dot_omega_bb/1, Integrator3/1
  UAV dynamics/1(lin_acc) -> Integrator1/1
  uT/1 -> UAV dynamics/1(uT)
  Integrator1/1 -> Linear_velocity/1, Integrator/1
  Integrator3/1 -> UAV dynamics/4(omega_bb), omega_bb/1
  UAV dynamics/2(dot_Rb) -> Integrator2/1, dot_Rb/1
  MATLAB Function1/1(Rb) -> Rb/1, UAV dynamics/3(Rb)
  Integrator2/1 -> MATLAB Function1/1(Rb_temp)

== system drones_simulation/Subsystem_Drone_4/Quadrotor dynamics ==
  uT : Inport
  tau_b : Inport  Port=2
  Integrator : Integrator  InitialCondition=x0_4
  Integrator1 : Integrator  InitialCondition=v0_4
  Integrator2 : Integrator  InitialCondition=[1 0 0; 0 1 0;0 0 1]
  Integrator3 : Integrator  InitialCondition=[0;0;0]
  MATLAB Function1 : MATLAB Function  TreatAsAtomicUnit=on
  UAV dynamics : MATLAB Function  TreatAsAtomicUnit=on
  Position : Outport
  Linear_velocity : Outport  Port=2
  Rb : Outport  Port=3
  dot_Rb : Outport  Port=4
  omega_bb : Outport  Port=5
  dot_omega_bb : Outport  Port=6
  wires:
  tau_b/1 -> UAV dynamics/2(tau_b)
  Integrator/1 -> Position/1
  UAV dynamics/3(ang_acc) -> dot_omega_bb/1, Integrator3/1
  UAV dynamics/1(lin_acc) -> Integrator1/1
  uT/1 -> UAV dynamics/1(uT)
  Integrator1/1 -> Linear_velocity/1, Integrator/1
  Integrator3/1 -> UAV dynamics/4(omega_bb), omega_bb/1
  UAV dynamics/2(dot_Rb) -> Integrator2/1, dot_Rb/1
  MATLAB Function1/1(Rb) -> Rb/1, UAV dynamics/3(Rb)
  Integrator2/1 -> MATLAB Function1/1(Rb_temp)

== matlab function drones_simulation/Safety_and_connectivity_Drone_1/MATLAB Function7 ==
  data: x_i input; v_i input; u_safe output; x_neighbors input; v_neighbors input; u_gtg input; gamma1 input; gamma2 input; Rs input; x_obs input; Rs_obs input; x_comm input; v_comm input; Rc input; max_acc input
function u_safe = QPsafety_i(x_i, v_i, x_neighbors, v_neighbors, u_gtg, ...
                             gamma1, gamma2, Rs, x_obs, Rs_obs, ...
                             x_comm, v_comm, Rc, max_acc)
%QPsafety_i  Filtra un comando nominale u_gtg con un QP + vincoli CBF/HOCBF.
%
% IDEA:
%   - Variabile ottimizzata: u (accelerazione 3D).
%   - Obiettivo: restare il più vicino possibile al comando nominale u_gtg.
%   - Vincoli: evitare ostacoli, evitare collisioni con vicini, mantenere connettività,
%              e non scendere sotto una quota minima (pavimento virtuale).
%
% FORMA QP (quadprog):
%   min_u   1/2 u' H u + f' u
%   s.t.    A u <= b -> vincoli per mantenere distanze e connettività
%           lb <= u <=  -> vincolo per non superare i limiti di
%           accelerazione
%
% 
%   I vincoli CBF usano una forma tipo "relative degree 2":
%       h_ddot + gamma1*h_dot + gamma2*h >= 0
%   che diventa un vincolo lineare in u (quindi compatibile con quadprog).

    %% (0) Dimensione del problema
    n_dims = 3;   % accelerazione 3D [ux; uy; uz]

    %% (1) Output di default
    % Se non serve filtrare o il QP non trova soluzione, almeno ritorniamo qualcosa.
    u_safe = u_gtg;

    %% (2) Constraints sull'accelerazione
    lb = -max_acc * ones(n_dims, 1);
    ub =  max_acc * ones(n_dims, 1);

    %% (3) Costo del QP: minimizza ||u - u_gtg||^2
    % quadprog minimizza: 1/2 u'Hu + f'u
    % Con H=2I e f=-2u_gtg, si ottiene (a costante vicina):
    %    1/2 u'(2I)u + (-2u_gtg)'u = u'u - 2u_gtg'u  ~ ||u-u_gtg||^2
    H_qp = 2 * eye(n_dims);
    f_qp = -2 * u_gtg;

    %% (4) Matrici vincoli lineari (si riempiono aggiungendo righe)
    % Ogni ostacolo/vicino genera un vincolo lineare del tipo: a^T u <= b
    A = zeros(0, n_dims);
    b = zeros(0, 1);

    %% (5) VINCOLI 1: Ostacoli statici (evitamento)
    % Barriera: h = ||p - p_obs||^2 - R^2 >= 0  (stai FUORI dalla sfera di raggio R)
    % Con doppio integratore: h_ddot = LfLfh + LgLfh*u
    % Vincolo HOCBF: h_ddot + gamma1*h_dot + gamma2*h >= 0
    n_obs = size(x_obs, 2);

    for k = 1:n_obs
        p_o = x_obs(:, k);      % posizione ostacolo k
        R_o = Rs_obs(k);        % raggio di sicurezza ostacolo k

        rel_p = x_i - p_o;      % posizione relativa
        rel_v = v_i;            % ostacolo fermo => v_rel = v_i

        dist_sq = norm(rel_p)^2;
        h      = dist_sq - R_o^2;
        h_dot  = 2 * rel_p' * rel_v;

        % Per h = ||rel_p||^2 - R^2:
        % LgLfh = 2*rel_p' (coefficiente davanti a u)
        % LfLfh = 2*||rel_v||^2 (termine noto, non dipende da u)
        LgLfh = 2 * rel_p';
        LfLfh = 2 * (rel_v' * rel_v);

        % quadprog vuole A*u <= b.
        % Dalla forma HOCBF si arriva a:  -(LgLfh) * u <= LfLfh + gamma1*h_dot + gamma2*h
        A = [A; -LgLfh];
        b = [b; (LfLfh + gamma1*h_dot + gamma2*h)];
    end

    %% (6) VINCOLI 2: Vicini (anti-collisione inter-agente)
    % Stesso tipo di barriera degli ostacoli, ma con posizione/velocità relative:
    %   h = ||p_i - p_j||^2 - Rs^2 >= 0  (distanza minima Rs)
    valid_cols = ~isnan(x_neighbors(1,:));
    n_max_neighbors = size(x_neighbors, 2);

    for k = 1:n_max_neighbors
        if valid_cols(k)
            p_j = x_neighbors(:, k);
            v_j = v_neighbors(:, k);

            rel_p = x_i - p_j;
            rel_v = v_i - v_j;

            dist_sq = norm(rel_p)^2;
            h      = dist_sq - Rs^2;
            h_dot  = 2 * rel_p' * rel_v;

            LgLfh = 2 * rel_p';
            LfLfh = 2 * (rel_v' * rel_v);

            A = [A; -LgLfh];
            b = [b; (LfLfh + gamma1*h_dot + gamma2*h)];
        end
    end

    %% (7) VINCOLI 3: Connettività / coesione (non allontanarsi oltre Rc)
    % Qui la barriera è "invertita" (stai DENTRO):
    %   h_c = Rc^2 - ||p_i - p_c||^2 >= 0  =>  ||p_i - p_c|| <= Rc
    valid_cols_comm = ~isnan(x_comm(1,:));
    n_max_comm = size(x_comm, 2);

    for k = 1:n_max_comm
        if valid_cols_comm(k)
            p_c = x_comm(:, k);
            v_c = v_comm(:, k);

            rel_p = x_i - p_c;
            rel_v = v_i - v_c;

            dist_sq = norm(rel_p)^2;

            h_c     = Rc^2 - dist_sq;
            h_dot_c = -2 * rel_p' * rel_v;

            % Segni diversi rispetto al caso "stai fuori":
            LgLfh_c = -2 * rel_p';
            LfLfh_c = -2 * (rel_v' * rel_v);

            % Anche qui si porta tutto in A*u <= b:
            A = [A; -LgLfh_c];
            b = [b; (LfLfh_c + gamma1*h_dot_c + gamma2*h_c)];
        end
    end

    %% (8) VINCOLO 4: Pavimento virtuale (z >= z_limit)
    % Barriera: h = z - z_limit >= 0
    % Con doppio integratore: h_dot = v_z, h_ddot = u_z
    z_limit = 0.1;

    z_pos = x_i(3);
    z_vel = v_i(3);

    h_floor     = z_pos - z_limit;
    h_dot_floor = z_vel;

    % Seleziona solo la componente u_z:
    LgLfh_floor = [0, 0, 1];
    LfLfh_floor = 0;

    % Vincolo: u_z + gamma1*v_z + gamma2*(z-z_limit) >= 0
    % => -u_z <= gamma1*v_z + gamma2*h_floor
    A = [A; -LgLfh_floor];   % [0 0 -1]
    b = [b; (LfLfh_floor + gamma1*h_dot_floor + gamma2*h_floor)];

    %% (9) Risoluzione del QP
    % Se non ci sono vincoli, restituisci direttamente u_gtg.
    if isempty(A)
        u_safe = u_gtg;
        return;
    end

    options = optimoptions('quadprog', ...
        'Algorithm', 'active-set', ...
        'Display', 'off');

    % Punto iniziale per il solver (warm start semplice)
    u0 = zeros(n_dims, 1);

    % Risolvi:
    [u_opt, ~, exitflag] = quadprog(H_qp, f_qp, A, b, [], [], lb, ub, u0, options);

    %% (10) Scelta finale dell'azione
    if exitflag == 1
        % Soluzione trovata: comando sicuro
        u_safe = u_opt;
    else
        % QP infeasible / non risolto: fallback conservativo (frenata)
        % u = -k*v riduce la velocità rapidamente
        u_safe = -2.0 * v_i;
    end
end

== matlab function drones_simulation/Safety_and_connectivity_Drone_2/MATLAB Function8 ==
  data: x_i input; v_i input; u_safe output; x_neighbors input; v_neighbors input; u_gtg input; gamma1 input; gamma2 input; Rs input; x_obs input; Rs_obs input; x_comm input; v_comm input; Rc input; max_acc input
function u_safe = QPsafety_i(x_i, v_i, x_neighbors, v_neighbors, u_gtg, ...
                             gamma1, gamma2, Rs, x_obs, Rs_obs, ...
                             x_comm, v_comm, Rc, max_acc)
%QPsafety_i  Filtra un comando nominale u_gtg con un QP + vincoli CBF/HOCBF.
%
% IDEA:
%   - Variabile ottimizzata: u (accelerazione 3D).
%   - Obiettivo: restare il più vicino possibile al comando nominale u_gtg.
%   - Vincoli: evitare ostacoli, evitare collisioni con vicini, mantenere connettività,
%              e non scendere sotto una quota minima (pavimento virtuale).
%
% FORMA QP (quadprog):
%   min_u   1/2 u' H u + f' u
%   s.t.    A u <= b -> vincoli per mantenere distanze e connettività
%           lb <= u <=  -> vincolo per non superare i limiti di
%           accelerazione
%
% 
%   I vincoli CBF usano una forma tipo "relative degree 2":
%       h_ddot + gamma1*h_dot + gamma2*h >= 0
%   che diventa un vincolo lineare in u (quindi compatibile con quadprog).

    %% (0) Dimensione del problema
    n_dims = 3;   % accelerazione 3D [ux; uy; uz]

    %% (1) Output di default
    % Se non serve filtrare o il QP non trova soluzione, almeno ritorniamo qualcosa.
    u_safe = u_gtg;

    %% (2) Constraints sull'accelerazione
    lb = -max_acc * ones(n_dims, 1);
    ub =  max_acc * ones(n_dims, 1);

    %% (3) Costo del QP: minimizza ||u - u_gtg||^2
    % quadprog minimizza: 1/2 u'Hu + f'u
    % Con H=2I e f=-2u_gtg, si ottiene (a costante vicina):
    %    1/2 u'(2I)u + (-2u_gtg)'u = u'u - 2u_gtg'u  ~ ||u-u_gtg||^2
    H_qp = 2 * eye(n_dims);
    f_qp = -2 * u_gtg;

    %% (4) Matrici vincoli lineari (si riempiono aggiungendo righe)
    % Ogni ostacolo/vicino genera un vincolo lineare del tipo: a^T u <= b
    A = zeros(0, n_dims);
    b = zeros(0, 1);

    %% (5) VINCOLI 1: Ostacoli statici (evitamento)
    % Barriera: h = ||p - p_obs||^2 - R^2 >= 0  (stai FUORI dalla sfera di raggio R)
    % Con doppio integratore: h_ddot = LfLfh + LgLfh*u
    % Vincolo HOCBF: h_ddot + gamma1*h_dot + gamma2*h >= 0
    n_obs = size(x_obs, 2);

    for k = 1:n_obs
        p_o = x_obs(:, k);      % posizione ostacolo k
        R_o = Rs_obs(k);        % raggio di sicurezza ostacolo k

        rel_p = x_i - p_o;      % posizione relativa
        rel_v = v_i;            % ostacolo fermo => v_rel = v_i

        dist_sq = norm(rel_p)^2;
        h      = dist_sq - R_o^2;
        h_dot  = 2 * rel_p' * rel_v;

        % Per h = ||rel_p||^2 - R^2:
        % LgLfh = 2*rel_p' (coefficiente davanti a u)
        % LfLfh = 2*||rel_v||^2 (termine noto, non dipende da u)
        LgLfh = 2 * rel_p';
        LfLfh = 2 * (rel_v' * rel_v);

        % quadprog vuole A*u <= b.
        % Dalla forma HOCBF si arriva a:  -(LgLfh) * u <= LfLfh + gamma1*h_dot + gamma2*h
        A = [A; -LgLfh];
        b = [b; (LfLfh + gamma1*h_dot + gamma2*h)];
    end

    %% (6) VINCOLI 2: Vicini (anti-collisione inter-agente)
    % Stesso tipo di barriera degli ostacoli, ma con posizione/velocità relative:
    %   h = ||p_i - p_j||^2 - Rs^2 >= 0  (distanza minima Rs)
    valid_cols = ~isnan(x_neighbors(1,:));
    n_max_neighbors = size(x_neighbors, 2);

    for k = 1:n_max_neighbors
        if valid_cols(k)
            p_j = x_neighbors(:, k);
            v_j = v_neighbors(:, k);

            rel_p = x_i - p_j;
            rel_v = v_i - v_j;

            dist_sq = norm(rel_p)^2;
            h      = dist_sq - Rs^2;
            h_dot  = 2 * rel_p' * rel_v;

            LgLfh = 2 * rel_p';
            LfLfh = 2 * (rel_v' * rel_v);

            A = [A; -LgLfh];
            b = [b; (LfLfh + gamma1*h_dot + gamma2*h)];
        end
    end

    %% (7) VINCOLI 3: Connettività / coesione (non allontanarsi oltre Rc)
    % Qui la barriera è "invertita" (stai DENTRO):
    %   h_c = Rc^2 - ||p_i - p_c||^2 >= 0  =>  ||p_i - p_c|| <= Rc
    valid_cols_comm = ~isnan(x_comm(1,:));
    n_max_comm = size(x_comm, 2);

    for k = 1:n_max_comm
        if valid_cols_comm(k)
            p_c = x_comm(:, k);
            v_c = v_comm(:, k);

            rel_p = x_i - p_c;
            rel_v = v_i - v_c;

            dist_sq = norm(rel_p)^2;

            h_c     = Rc^2 - dist_sq;
            h_dot_c = -2 * rel_p' * rel_v;

            % Segni diversi rispetto al caso "stai fuori":
            LgLfh_c = -2 * rel_p';
            LfLfh_c = -2 * (rel_v' * rel_v);

            % Anche qui si porta tutto in A*u <= b:
            A = [A; -LgLfh_c];
            b = [b; (LfLfh_c + gamma1*h_dot_c + gamma2*h_c)];
        end
    end

    %% (8) VINCOLO 4: Pavimento virtuale (z >= z_limit)
    % Barriera: h = z - z_limit >= 0
    % Con doppio integratore: h_dot = v_z, h_ddot = u_z
    z_limit = 0.1;

    z_pos = x_i(3);
    z_vel = v_i(3);

    h_floor     = z_pos - z_limit;
    h_dot_floor = z_vel;

    % Seleziona solo la componente u_z:
    LgLfh_floor = [0, 0, 1];
    LfLfh_floor = 0;

    % Vincolo: u_z + gamma1*v_z + gamma2*(z-z_limit) >= 0
    % => -u_z <= gamma1*v_z + gamma2*h_floor
    A = [A; -LgLfh_floor];   % [0 0 -1]
    b = [b; (LfLfh_floor + gamma1*h_dot_floor + gamma2*h_floor)];

    %% (9) Risoluzione del QP
    % Se non ci sono vincoli, restituisci direttamente u_gtg.
    if isempty(A)
        u_safe = u_gtg;
        return;
    end

    options = optimoptions('quadprog', ...
        'Algorithm', 'active-set', ...
        'Display', 'off');

    % Punto iniziale per il solver (warm start semplice)
    u0 = zeros(n_dims, 1);

    % Risolvi:
    [u_opt, ~, exitflag] = quadprog(H_qp, f_qp, A, b, [], [], lb, ub, u0, options);

    %% (10) Scelta finale dell'azione
    if exitflag == 1
        % Soluzione trovata: comando sicuro
        u_safe = u_opt;
    else
        % QP infeasible / non risolto: fallback conservativo (frenata)
        % u = -k*v riduce la velocità rapidamente
        u_safe = -2.0 * v_i;
    end
end

== matlab function drones_simulation/Safety_and_connectivity_Drone_3/MATLAB Function9 ==
  data: x_i input; v_i input; u_safe output; x_neighbors input; v_neighbors input; u_gtg input; gamma1 input; gamma2 input; Rs input; x_obs input; Rs_obs input; x_comm input; v_comm input; Rc input; max_acc input
function u_safe = QPsafety_i(x_i, v_i, x_neighbors, v_neighbors, u_gtg, ...
                             gamma1, gamma2, Rs, x_obs, Rs_obs, ...
                             x_comm, v_comm, Rc, max_acc)
%QPsafety_i  Filtra un comando nominale u_gtg con un QP + vincoli CBF/HOCBF.
%
% IDEA:
%   - Variabile ottimizzata: u (accelerazione 3D).
%   - Obiettivo: restare il più vicino possibile al comando nominale u_gtg.
%   - Vincoli: evitare ostacoli, evitare collisioni con vicini, mantenere connettività,
%              e non scendere sotto una quota minima (pavimento virtuale).
%
% FORMA QP (quadprog):
%   min_u   1/2 u' H u + f' u
%   s.t.    A u <= b -> vincoli per mantenere distanze e connettività
%           lb <= u <=  -> vincolo per non superare i limiti di
%           accelerazione
%
% 
%   I vincoli CBF usano una forma tipo "relative degree 2":
%       h_ddot + gamma1*h_dot + gamma2*h >= 0
%   che diventa un vincolo lineare in u (quindi compatibile con quadprog).

    %% (0) Dimensione del problema
    n_dims = 3;   % accelerazione 3D [ux; uy; uz]

    %% (1) Output di default
    % Se non serve filtrare o il QP non trova soluzione, almeno ritorniamo qualcosa.
    u_safe = u_gtg;

    %% (2) Constraints sull'accelerazione
    lb = -max_acc * ones(n_dims, 1);
    ub =  max_acc * ones(n_dims, 1);

    %% (3) Costo del QP: minimizza ||u - u_gtg||^2
    % quadprog minimizza: 1/2 u'Hu + f'u
    % Con H=2I e f=-2u_gtg, si ottiene (a costante vicina):
    %    1/2 u'(2I)u + (-2u_gtg)'u = u'u - 2u_gtg'u  ~ ||u-u_gtg||^2
    H_qp = 2 * eye(n_dims);
    f_qp = -2 * u_gtg;

    %% (4) Matrici vincoli lineari (si riempiono aggiungendo righe)
    % Ogni ostacolo/vicino genera un vincolo lineare del tipo: a^T u <= b
    A = zeros(0, n_dims);
    b = zeros(0, 1);

    %% (5) VINCOLI 1: Ostacoli statici (evitamento)
    % Barriera: h = ||p - p_obs||^2 - R^2 >= 0  (stai FUORI dalla sfera di raggio R)
    % Con doppio integratore: h_ddot = LfLfh + LgLfh*u
    % Vincolo HOCBF: h_ddot + gamma1*h_dot + gamma2*h >= 0
    n_obs = size(x_obs, 2);

    for k = 1:n_obs
        p_o = x_obs(:, k);      % posizione ostacolo k
        R_o = Rs_obs(k);        % raggio di sicurezza ostacolo k

        rel_p = x_i - p_o;      % posizione relativa
        rel_v = v_i;            % ostacolo fermo => v_rel = v_i

        dist_sq = norm(rel_p)^2;
        h      = dist_sq - R_o^2;
        h_dot  = 2 * rel_p' * rel_v;

        % Per h = ||rel_p||^2 - R^2:
        % LgLfh = 2*rel_p' (coefficiente davanti a u)
        % LfLfh = 2*||rel_v||^2 (termine noto, non dipende da u)
        LgLfh = 2 * rel_p';
        LfLfh = 2 * (rel_v' * rel_v);

        % quadprog vuole A*u <= b.
        % Dalla forma HOCBF si arriva a:  -(LgLfh) * u <= LfLfh + gamma1*h_dot + gamma2*h
        A = [A; -LgLfh];
        b = [b; (LfLfh + gamma1*h_dot + gamma2*h)];
    end

    %% (6) VINCOLI 2: Vicini (anti-collisione inter-agente)
    % Stesso tipo di barriera degli ostacoli, ma con posizione/velocità relative:
    %   h = ||p_i - p_j||^2 - Rs^2 >= 0  (distanza minima Rs)
    valid_cols = ~isnan(x_neighbors(1,:));
    n_max_neighbors = size(x_neighbors, 2);

    for k = 1:n_max_neighbors
        if valid_cols(k)
            p_j = x_neighbors(:, k);
            v_j = v_neighbors(:, k);

            rel_p = x_i - p_j;
            rel_v = v_i - v_j;

            dist_sq = norm(rel_p)^2;
            h      = dist_sq - Rs^2;
            h_dot  = 2 * rel_p' * rel_v;

            LgLfh = 2 * rel_p';
            LfLfh = 2 * (rel_v' * rel_v);

            A = [A; -LgLfh];
            b = [b; (LfLfh + gamma1*h_dot + gamma2*h)];
        end
    end

    %% (7) VINCOLI 3: Connettività / coesione (non allontanarsi oltre Rc)
    % Qui la barriera è "invertita" (stai DENTRO):
    %   h_c = Rc^2 - ||p_i - p_c||^2 >= 0  =>  ||p_i - p_c|| <= Rc
    valid_cols_comm = ~isnan(x_comm(1,:));
    n_max_comm = size(x_comm, 2);

    for k = 1:n_max_comm
        if valid_cols_comm(k)
            p_c = x_comm(:, k);
            v_c = v_comm(:, k);

            rel_p = x_i - p_c;
            rel_v = v_i - v_c;

            dist_sq = norm(rel_p)^2;

            h_c     = Rc^2 - dist_sq;
            h_dot_c = -2 * rel_p' * rel_v;

            % Segni diversi rispetto al caso "stai fuori":
            LgLfh_c = -2 * rel_p';
            LfLfh_c = -2 * (rel_v' * rel_v);

            % Anche qui si porta tutto in A*u <= b:
            A = [A; -LgLfh_c];
            b = [b; (LfLfh_c + gamma1*h_dot_c + gamma2*h_c)];
        end
    end

    %% (8) VINCOLO 4: Pavimento virtuale (z >= z_limit)
    % Barriera: h = z - z_limit >= 0
    % Con doppio integratore: h_dot = v_z, h_ddot = u_z
    z_limit = 0.1;

    z_pos = x_i(3);
    z_vel = v_i(3);

    h_floor     = z_pos - z_limit;
    h_dot_floor = z_vel;

    % Seleziona solo la componente u_z:
    LgLfh_floor = [0, 0, 1];
    LfLfh_floor = 0;

    % Vincolo: u_z + gamma1*v_z + gamma2*(z-z_limit) >= 0
    % => -u_z <= gamma1*v_z + gamma2*h_floor
    A = [A; -LgLfh_floor];   % [0 0 -1]
    b = [b; (LfLfh_floor + gamma1*h_dot_floor + gamma2*h_floor)];

    %% (9) Risoluzione del QP
    % Se non ci sono vincoli, restituisci direttamente u_gtg.
    if isempty(A)
        u_safe = u_gtg;
        return;
    end

    options = optimoptions('quadprog', ...
        'Algorithm', 'active-set', ...
        'Display', 'off');

    % Punto iniziale per il solver (warm start semplice)
    u0 = zeros(n_dims, 1);

    % Risolvi:
    [u_opt, ~, exitflag] = quadprog(H_qp, f_qp, A, b, [], [], lb, ub, u0, options);

    %% (10) Scelta finale dell'azione
    if exitflag == 1
        % Soluzione trovata: comando sicuro
        u_safe = u_opt;
    else
        % QP infeasible / non risolto: fallback conservativo (frenata)
        % u = -k*v riduce la velocità rapidamente
        u_safe = -2.0 * v_i;
    end
end
